simulink model "problem_4"  (R2020b)
settings: Solver=VariableStepAuto  StartTime=0.0  StopTime=10.0  RelTol=1e-3
settings Model: Creator=k.Raviteja  LastModifiedBy=k.Raviteja

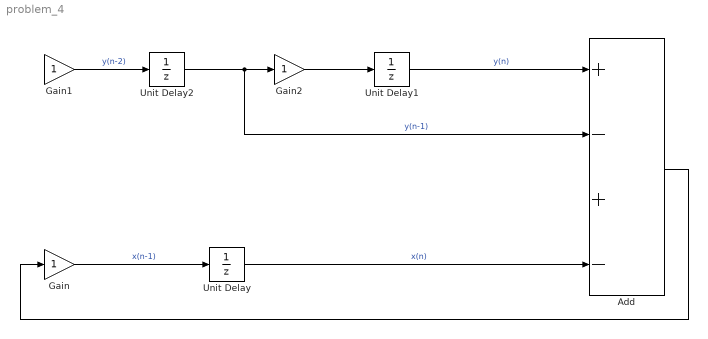
== system problem_4 ==
  Add : Sum  Inputs=+-+-
  Gain : Gain
  Gain1 : Gain
  Gain2 : Gain
  Unit Delay : UnitDelay  SampleTime=-1  HasFrameUpgradeWarning=on
  Unit Delay1 : UnitDelay  SampleTime=-1  HasFrameUpgradeWarning=on
  Unit Delay2 : UnitDelay  SampleTime=-1  HasFrameUpgradeWarning=on
  wires:
  Unit Delay2/1 -> Add/2, Gain2/1  "y(n-1)"
  Unit Delay1/1 -> Add/1  "y(n)"
  Gain1/1 -> Unit Delay2/1  "y(n-2)"
  Unit Delay/1 -> Add/4  "x(n)"
  Gain/1 -> Unit Delay/1  "x(n-1)"
  Gain2/1 -> Unit Delay1/1
  Add/1 -> Gain/1
  ? -> Gain1/1
